simulink model "HW1 (2)"  (R2018b)
settings: Solver=VariableStepAuto  StartTime=0.0  StopTime=20  RelTol=1e-3
settings Model: Creator=Boris  LastModifiedBy=Boris
settings DataIOCC: ReturnWorkspaceOutputs=on

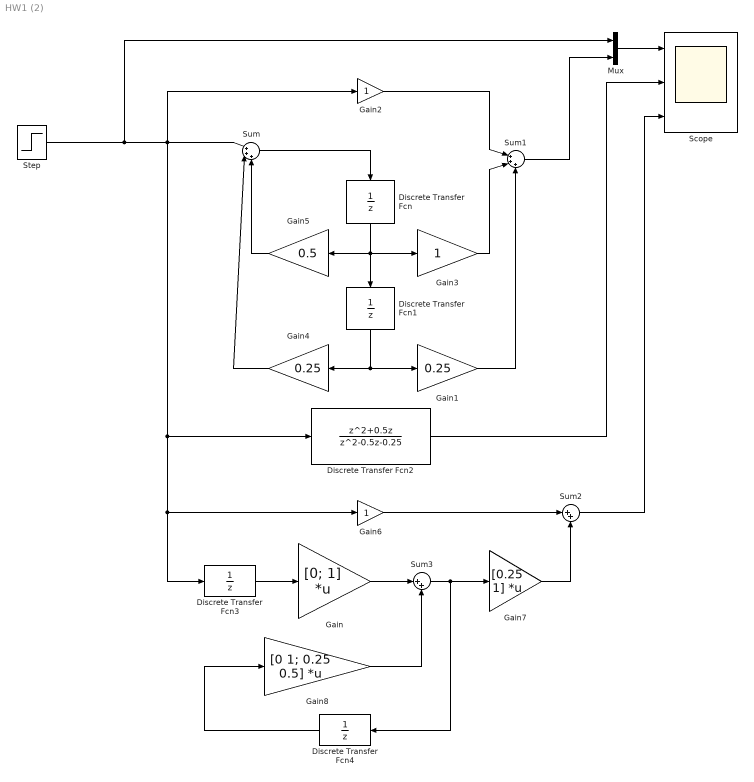
== system HW1 (2) ==
  Discrete Transfer Fcn{,1,3..4} (4 alike) : DiscreteTransferFcn  Denominator=[1 0]
  Discrete Transfer Fcn2 : DiscreteTransferFcn  Numerator=[1 0.5 0]  Denominator=[1 -0.5 -0.25]
  Gain : Gain  Gain=[0; 1]  Multiplication=Matrix(K*u)
  Gain1 : Gain  Gain=0.25
  Gain2 : Gain
  Gain3 : Gain
  Gain4 : Gain  Gain=0.25
  Gain5 : Gain  Gain=0.5
  Gain6 : Gain
  Gain7 : Gain  Gain=[0.25 1]  Multiplication=Matrix(K*u)
  Gain8 : Gain  Gain=[0 1; 0.25 0.5]  Multiplication=Matrix(K*u)
  Mux : Mux  Inputs=2
  Scope : Scope  NumInputPorts=3
  Step : Step  Time=0  SampleTime=0
  Sum : Sum  Inputs=|+++
  Sum1 : Sum  Inputs=|+++
  Sum2 : Sum  Inputs=|++
  Sum3 : Sum  Inputs=|++
  wires:
  Discrete Transfer Fcn1/1 -> Gain4/1, Gain1/1
  Discrete Transfer Fcn/1 -> Gain5/1, Gain3/1, Discrete Transfer Fcn1/1
  Gain4/1 -> Sum/2
  Gain5/1 -> Sum/3
  Sum/1 -> Discrete Transfer Fcn/1
  Gain2/1 -> Sum1/1
  Gain3/1 -> Sum1/2
  Gain1/1 -> Sum1/3
  Step/1 -> Mux/1, Discrete Transfer Fcn3/1, Gain6/1, Discrete Transfer Fcn2/1, Gain2/1, Sum/1
  Sum1/1 -> Mux/2
  Discrete Transfer Fcn2/1 -> Scope/2
  Mux/1 -> Scope/1
  Discrete Transfer Fcn3/1 -> Gain/1
  Discrete Transfer Fcn4/1 -> Gain8/1
  Gain8/1 -> Sum3/2
  Gain/1 -> Sum3/1
  Sum3/1 -> Discrete Transfer Fcn4/1, Gain7/1
  Gain7/1 -> Sum2/2
  Gain6/1 -> Sum2/1
  Sum2/1 -> Scope/3
